simulink model "velocityp2"  (R2023a)
settings: Solver=VariableStepAuto  StartTime=0.0  StopTime=10.0  RelTol=1e-3
settings Model: Creator=mluser  LastModifiedBy=mluser

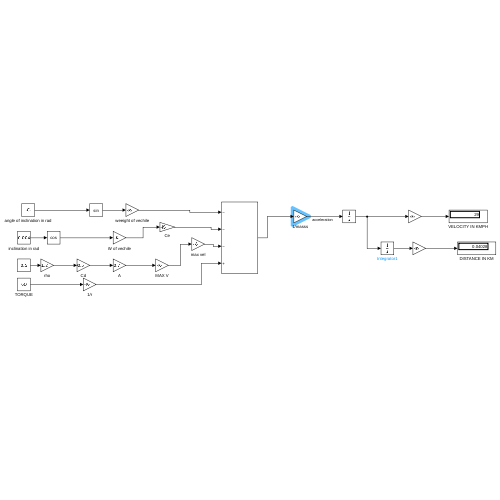
[thumbnail: Simulink's stored preview of the top-level diagram]
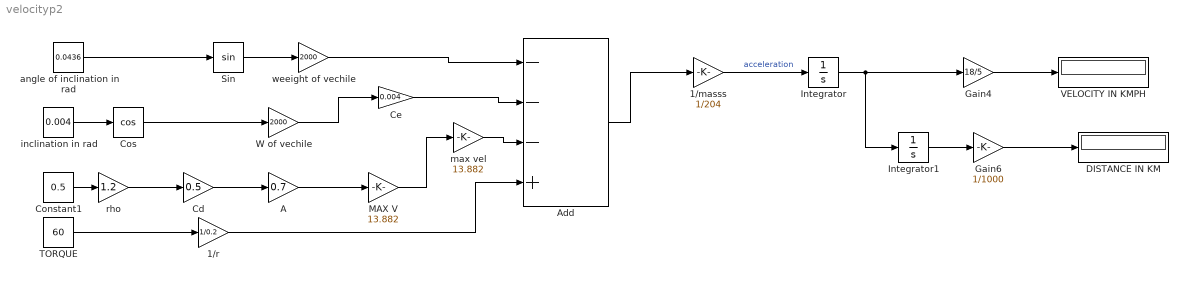
== system velocityp2 ==
  1/masss : Gain  Gain=1/204
  1/r : Gain  Gain=1/0.2
  A : Gain  Gain=0.7
  Add : Sum  Inputs=---+
  Cd : Gain  Gain=0.5
  Ce : Gain  Gain=0.004
  Constant1 : Constant  Value=0.5
  Cos : Trigonometry  Operator=cos
  DISTANCE IN KM : Display
  Gain4 : Gain  Gain=18/5
  Gain6 : Gain  Gain=1/1000
  Integrator : Integrator
  Integrator1 : Integrator
  MAX V : Gain  Gain=13.882
  Sin : Trigonometry
  TORQUE : Constant  Value=60
  VELOCITY IN KMPH : Display
  W of vechile : Gain  Gain=2000
  angle of inclination in rad : Constant  Value=0.0436
  inclination in rad : Constant  Value=0.004
  max vel : Gain  Gain=13.882
  rho : Gain  Gain=1.2
  weeight of vechile : Gain  Gain=2000
  wires:
  angle of inclination in rad/1 -> Sin/1
  Sin/1 -> weeight of vechile/1
  inclination in rad/1 -> Cos/1
  Constant1/1 -> rho/1
  rho/1 -> Cd/1
  Cd/1 -> A/1
  A/1 -> MAX V/1
  TORQUE/1 -> 1/r/1
  1/masss/1 -> Integrator/1  "acceleration"
  Integrator/1 -> Integrator1/1, Gain4/1
  Integrator1/1 -> Gain6/1
  Gain4/1 -> VELOCITY IN KMPH/1
  weeight of vechile/1 -> Add/1
  Cos/1 -> W of vechile/1
  MAX V/1 -> max vel/1
  Add/1 -> 1/masss/1
  Gain6/1 -> DISTANCE IN KM/1
  W of vechile/1 -> Ce/1
  Ce/1 -> Add/2
  max vel/1 -> Add/3
  1/r/1 -> Add/4
